simulink model "mBraccioHW"  (R2021a)
settings: Solver=FixedStepAuto  StartTime=0.0  StopTime=inf  RelTol=1e-3  EnableMultiTasking=on
InitFcn:
  | % oJointBase      = classes.Joint(deg2rad(0)-pi/2, deg2rad(180)-pi/2);
  | % oJointShoulder  = classes.Joint(deg2rad(15)-pi/2, deg2rad(165)-pi/2);
  | % oJointElbow     = classes.Joint(deg2rad(0)-pi/2, deg2rad(180)-pi/2);
  | % oJointPitch     = classes.Joint(deg2rad(0)-pi/2, deg2rad(180)-pi/2);
  | % oJointWrist     = classes.Joint(deg2rad(0)-pi/2, deg2rad(180)-pi/2);
  | 
  | % oLinkGround     = classes.Link(70);
  | % oLinkArm        = classes.Link(125);
  | % oLinkForearm    = classes.Link(125);
  | % oLinkHand       = classes.Link(185);
undefined symbols (not defined in the file): adHome6deg, adHome6rad, adWS
libraries: arduinolib x13, aerolibconvert2 x2
settings Model: SILPILModeSetting=veronly  ExtModeTrigDuration=2  Creator=angelo  LastModifiedBy=angelo
settings OptimizationCC: EnhancedBackFolding=on  PassReuseOutputArgsAs=Individual arguments  ZeroExternalMemoryAtStartup=off  ZeroInternalMemoryAtStartup=off  MaxStackSize=64  OptimizeBlockOrder=speed  DifferentSizesBufferReuse=on  OptimizationCustomize=off  EfficientTunableParamExpr=on
settings DebuggingCC: ParameterTunabilityLossMsg=error
settings HardwareCC: ProdBitPerInt=16  ProdBitPerPointer=16  ProdBitPerSizeT=16  ProdBitPerPtrDiffT=16  ProdLargestAtomicFloat=None  ProdWordSize=8  ProdHWDeviceType=Atmel->AVR
settings SFSimCC: MATLABDynamicMemAlloc=off
settings RTWCC: SystemTargetFile=ert.tlc  HardwareBoard=Arduino Mega 2560  TemplateMakefile=ert_default_tmf  Toolchain=Arduino AVR  BuildConfiguration=Faster Runs
settings CodeAppCC: ForceParamTrailComments=on  IgnoreCustomStorageClasses=off  OperatorAnnotations=on  SimulinkDataObjDesc=on  SFDataObjDesc=on  InsertBlockDesc=on
settings ERTTargetCC: SupportContinuousTime=on  SupportVariableSizeSignals=on  ExtModeStaticAllocSize=2048

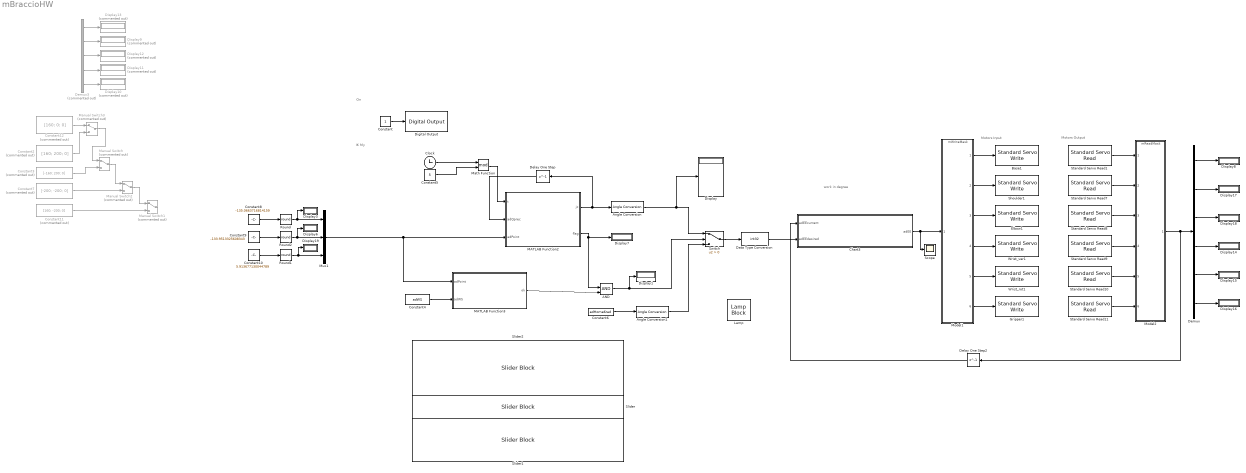
== system mBraccioHW ==
  note: On
  note: IK My
  note: work in degree
  note: Motors Input
  note: Motors Output
  AND : Logic  IconShape=distinctive  AllPortsSameDT=off  OutDataTypeStr=boolean
  Angle Conversion : aerolibconvert2/Angle Conversion  IU=rad  OU=deg
  Angle Conversion1 : aerolibconvert2/Angle Conversion  IU=rad  OU=deg
  Base1 : arduinolib/Standard Servo Write  pinNumber=11  ServoIndex=0  blockPlatform=ARDUINO
  Chart3 : Stateflow chart  TreatAsAtomicUnit=on  SystemSampleTime=0.02
  Clock : Clock
  Constant : Constant
  Constant10 : Constant  Value=5.913677130044789
  Constant11 : Constant  Commented=on  Value=[160; -200; 0]
  Constant12 : Constant  Commented=on  Value=[160; 0; 0]
  Constant2 : Constant  Commented=on  Value=[160; 200; 0]
  Constant3 : Constant  Commented=on  Value=[-160; 200; 0]
  Constant4 : Constant  Value=adWS
  Constant5 : Constant  Value=5
  Constant6 : Constant  Value=adHome6rad
  Constant7 : Constant  Commented=on  Value=[-200; -200; 0]
  Constant8 : Constant  Value=-135.0663716814159
  Constant9 : Constant  Value=-133.9513325608343
  Data Type Conversion : DataTypeConversion  OutDataTypeStr=int32  RndMeth=Round
  Delay One Step : Delay  DelayLength=1  InitialCondition=adHome6rad  SampleTime=0.02
  Delay One Step2 : Delay  DelayLength=1  InitialCondition=adHome6deg
  Demux : Demux  Outputs=6
  Demux3 : Demux  Commented=on  Outputs=5
  Digital Output : arduinolib/Digital Output  pinNumber=12  Direction=output  blockPlatform=arduino
  Display{,1,3,6..8,14..19} (12 alike) : Display
  Display{9..13} (5 alike) : Display  Commented=on
  Elbow1 : arduinolib/Standard Servo Write  pinNumber=9  ServoIndex=1  blockPlatform=ARDUINO
  Gripper1 : arduinolib/Standard Servo Write  pinNumber=3  ServoIndex=2  blockPlatform=ARDUINO
  Lamp : LampBlock
  MATLAB Function2 : MATLAB Function  TreatAsAtomicUnit=on  SystemSampleTime=0.02
  MATLAB Function3 : MATLAB Function  TreatAsAtomicUnit=on  SystemSampleTime=0.02
  Manual Switch{,1..3} (4 alike) : ManualSwitch  Commented=on
  Math Function : Math  Operator=mod  SaturateOnIntegerOverflow=on
  Model1 : ModelReference  ModelNameDialog=mWriteMask.slx  SimulationMode=Normal  ModelReferenceVersion=1.3
  Model2 : ModelReference  ModelNameDialog=mReadMask.slx  SimulationMode=Normal  ModelReferenceVersion=1.4
  Mux1 : Mux  Inputs=3
  Round : Rounding  Operator=round
  Round1 : Rounding  Operator=round
  Round2 : Rounding  Operator=round
  Scope : Scope
  Shoulder1 : arduinolib/Standard Servo Write  pinNumber=10  ServoIndex=3  blockPlatform=ARDUINO
  Slider : SliderBlock  LabelPosition=Hide  ScaleMin=-400  ScaleMax=+400
  Slider1 : SliderBlock  LabelPosition=Hide  ScaleMin=-400  ScaleMax=400
  Slider2 : SliderBlock  LabelPosition=Hide  ScaleMin=-400  ScaleMax=400
  Standard Servo Read1 : arduinolib/Standard Servo Read  pinNumber=11  SampleTime=0.02  ServoIndex=0  blockPlatform=ARDUINO
      settings: SourceProductBaseCode=ARDUINO
  Standard Servo Read10 : arduinolib/Standard Servo Read  pinNumber=5  SampleTime=0.02  ServoIndex=4  blockPlatform=ARDUINO
      settings: SourceProductBaseCode=ARDUINO
  Standard Servo Read11 : arduinolib/Standard Servo Read  pinNumber=3  SampleTime=0.02  ServoIndex=2  blockPlatform=ARDUINO
      settings: SourceProductBaseCode=ARDUINO
  Standard Servo Read7 : arduinolib/Standard Servo Read  pinNumber=10  SampleTime=0.02  ServoIndex=3  blockPlatform=ARDUINO
      settings: SourceProductBaseCode=ARDUINO
  Standard Servo Read8 : arduinolib/Standard Servo Read  pinNumber=9  SampleTime=0.02  ServoIndex=1  blockPlatform=ARDUINO
      settings: SourceProductBaseCode=ARDUINO
  Standard Servo Read9 : arduinolib/Standard Servo Read  pinNumber=6  SampleTime=0.02  ServoIndex=5  blockPlatform=ARDUINO
      settings: SourceProductBaseCode=ARDUINO
  Switch : Switch  Criteria=u2 > Threshold
  Wrist_rot1 : arduinolib/Standard Servo Write  pinNumber=5  ServoIndex=4  blockPlatform=ARDUINO
  Wrist_ver1 : arduinolib/Standard Servo Write  pinNumber=6  ServoIndex=5  blockPlatform=ARDUINO
  wires:
  Constant/1 -> Digital Output/1
  Demux3/1 -> Display13/1
  Demux3/3 -> Display12/1
  Demux3/5 -> Display10/1
  Demux3/2 -> Display9/1
  Demux3/4 -> Display11/1
  Chart3/1(adEE) -> Model1/1, Scope/1
  Delay One Step2/1 -> Chart3/1(adEEcurrent)
  MATLAB Function2/2(flag) -> AND/1, Display7/1
  MATLAB Function2/1(jc) -> Angle Conversion/1, Delay One Step/1
  Constant4/1 -> MATLAB Function3/2(adWS)
  MATLAB Function3/1(ok) -> AND/2
  AND/1 -> Switch/2, Display1/1
  Constant6/1 -> Angle Conversion1/1
  Angle Conversion1/1 -> Switch/3
  Clock/1 -> Math Function/1
  Constant5/1 -> Math Function/2
  Math Function/1 -> MATLAB Function2/1(t)
  Delay One Step/1 -> MATLAB Function2/2(adQprec)
  Constant8/1 -> Round/1
  Constant9/1 -> Round2/1
  Constant10/1 -> Round1/1
  Constant3/1 -> Manual Switch/2
  Manual Switch/1 -> Manual Switch2/1
  Constant7/1 -> Manual Switch2/2
  Manual Switch2/1 -> Manual Switch1/1
  Constant11/1 -> Manual Switch1/2
  Round1/1 -> Display19/1, Mux1/3
  Round/1 -> Display3/1, Mux1/1
  Constant12/1 -> Manual Switch3/1
  Constant2/1 -> Manual Switch3/2
  Manual Switch3/1 -> Manual Switch/1
  Demux/2 -> Display17/1
  Demux/3 -> Display18/1
  Demux/1 -> Display8/1
  Demux/5 -> Display15/1
  Demux/4 -> Display14/1
  Round2/1 -> Display6/1, Mux1/2
  Mux1/1 -> MATLAB Function3/1(adPoint), MATLAB Function2/3(adPoint)
  Demux/6 -> Display16/1
  Angle Conversion/1 -> Display/1, Switch/1
  Switch/1 -> Data Type Conversion/1
  Data Type Conversion/1 -> Chart3/2(adEEdesired)
  Model1/1 -> Base1/1
  Model1/2 -> Shoulder1/1
  Model1/3 -> Elbow1/1
  Model1/4 -> Wrist_ver1/1
  Model1/5 -> Wrist_rot1/1
  Model1/6 -> Gripper1/1
  Standard Servo Read1/1 -> Model2/1
  Standard Servo Read7/1 -> Model2/2
  Standard Servo Read8/1 -> Model2/3
  Standard Servo Read9/1 -> Model2/4
  Standard Servo Read10/1 -> Model2/5
  Standard Servo Read11/1 -> Model2/6
  Model2/1 -> Delay One Step2/1, Demux/1

== matlab function mBraccioHW/MATLAB Function2 ==
  data: t input; adQprec input; adPoint input; jc output; flag output
function [jc, flag] = ikin(t, adQprec, adPoint)
if(t ~= 0)
    flag  	= true;
    jc      = adQprec;
    return;
end

% Joints definition
oJointBase      = classes.Joint(deg2rad(0)-pi/2, deg2rad(180)-pi/2);
oJointShoulder  = classes.Joint(deg2rad(15)-pi/2, deg2rad(165)-pi/2);
oJointElbow     = classes.Joint(deg2rad(0)-pi/2, deg2rad(180)-pi/2);
oJointPitch     = classes.Joint(deg2rad(0)-pi/2, deg2rad(180)-pi/2);
oJointWrist     = classes.Joint(deg2rad(0)-pi/2, deg2rad(180)-pi/2);

% Liks definition
%oLinkGround     = classes.Link(70);
%oLinkArm        = classes.Link(125);
%oLinkForearm    = classes.Link(125);
%oLinkHand       = classes.Link(185);

oLinkGround     = classes.Link(74);
oLinkArm        = classes.Link(125);
oLinkForearm    = classes.Link(125);
oLinkHand       = classes.Link(195);

% Braccio definition
oBraccio        = classes.Robot5Dof(oJointBase, oJointShoulder,     ...
                                    oJointElbow, oJointPitch,       ... 
                                    oJointWrist, oLinkGround,       ...
                                    oLinkArm, oLinkForearm,         ...
                                    oLinkHand);

% IKIN computation
[bOK, adQ]      = oBraccio.IKIN(adPoint);

% Output
jc              = [adQ + pi/2; 0; deg2rad(70)];
flag            = bOK;
end

== stateflow chart mBraccioHW/Chart3 ==
  settings: executeAtInitialization=1
  state First
    during:
    adEE = [
    nextStep(adEEcurrent(1), adEEdesired(1));
    nextStep(adEEcurrent(2), adEEdesired(2));
    nextStep(adEEcurrent(3), adEEdesired(3));
    nextStep(adEEcurrent(4), adEEdesired(4));
    nextStep(adEEcurrent(5), adEEdesired(5));
    nextStep(adEEcurrent(6), adEEdesired(6)) ];
  (default) -> First
  data: current function_input; desired function_input; v function_output; adEEcurrent input; adEE output; adEEdesired input
  function v = nextStep(current, desired):
    | function v = nextStep(current, desired)
    | if (current < desired)
    |     current = current + 1;
    | end
    | 
    | if (current > desired)
    |     current = current - 1;
    | end
    | 
    | v = current;
    | end

== matlab function mBraccioHW/MATLAB Function3 ==
  data: adPoint input; ok output; adWS input
function ok = verifierWS(adPoint, adWS)
ok = functions.isInsideWorkspace(adPoint, adWS(1), adWS(2), adWS(3));
end
